simulink model "Diagramas de bloques de un reactor quimico"  (R2018a)
settings: Solver=VariableStepAuto  StartTime=0.0  StopTime=500  RelTol=1e-3
settings Model: Creator=Paulo  LastModifiedBy=Paulo

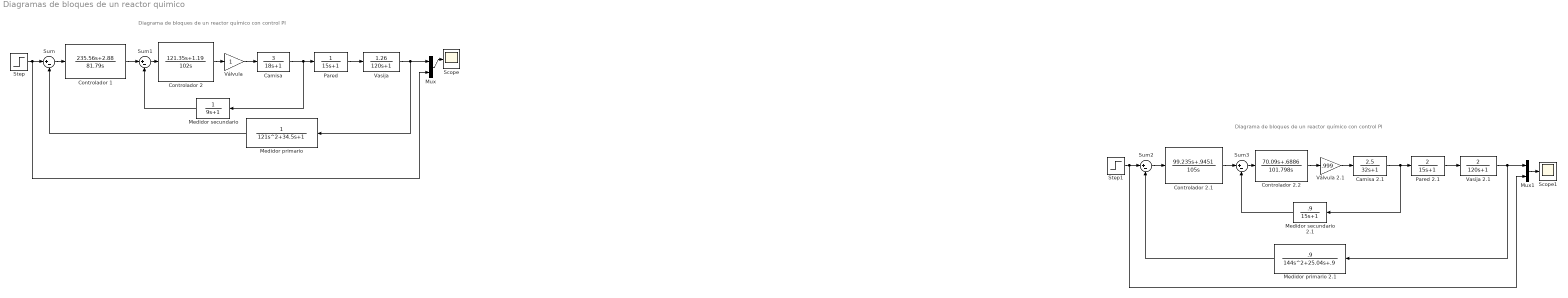
== system Diagramas de bloques de un reactor quimico ==
  note: Diagrama de bloques de un reactor químico con control PI
  note: Diagrama de bloques de un reactor químico con control PI
  Camisa : TransferFcn  Numerator=[3]  Denominator=[18 1]
  Camisa 2.1 : TransferFcn  Numerator=[2.5]  Denominator=[32 1]
  Controlador 1 : TransferFcn  Numerator=[235.56 2.88]  Denominator=[81.79 0]
  Controlador 2 : TransferFcn  Numerator=[121.35 1.19]  Denominator=[102 0]
  "Controlador 2.1 " : TransferFcn  Numerator=[99.235 .9451]  Denominator=[105 0]
  Controlador 2.2 : TransferFcn  Numerator=[70.09 .6886]  Denominator=[101.798 0]
  Medidor primario : TransferFcn  Denominator=[121 34.5 1]
  Medidor primario 2.1 : TransferFcn  Numerator=[.9]  Denominator=[144 25.04 .9]
  Medidor secundario : TransferFcn  Denominator=[9 1]
  Medidor secundario 2.1 : TransferFcn  Numerator=[.9]  Denominator=[15 1]
  Mux : Mux  Inputs=2
  Mux1 : Mux  Inputs=2
  Pared : TransferFcn  Denominator=[15 1]
  Pared 2.1 : TransferFcn  Numerator=[2]  Denominator=[15 1]
  Scope : Scope
  Scope1 : Scope
  Step : Step  Time=0  SampleTime=0
  Step1 : Step  Time=0  SampleTime=0
  Sum{,1..3} (4 alike) : Sum  Inputs=|+-
  Vasija : TransferFcn  Numerator=[1.26]  Denominator=[120 1]
  Vasija 2.1 : TransferFcn  Numerator=[2]  Denominator=[120 1]
  Válvula : Gain
  Válvula 2.1 : Gain  Gain=.999
  wires:
  Step/1 -> Sum/1, Mux/2
  Sum/1 -> Controlador 1/1
  Camisa/1 -> Medidor secundario/1, Pared/1
  Medidor secundario/1 -> Sum1/2
  Válvula/1 -> Camisa/1
  Pared/1 -> Vasija/1
  Vasija/1 -> Mux/1, Medidor primario/1
  Medidor primario/1 -> Sum/2
  Mux/1 -> Scope/1
  Controlador 1/1 -> Sum1/1
  Sum1/1 -> Controlador 2/1
  Controlador 2/1 -> Válvula/1
  Mux1/1 -> Scope1/1
  Camisa 2.1/1 -> Medidor secundario 2.1/1, Pared 2.1/1
  Medidor primario 2.1/1 -> Sum2/2
  Medidor secundario 2.1/1 -> Sum3/2
  Vasija 2.1/1 -> Mux1/1, Medidor primario 2.1/1
  Step1/1 -> Sum2/1, Mux1/2
  Pared 2.1/1 -> Vasija 2.1/1
  Válvula 2.1/1 -> Camisa 2.1/1
  Controlador 2.2/1 -> Válvula 2.1/1
  Sum3/1 -> Controlador 2.2/1
  Sum2/1 -> "Controlador 2.1 "/1
  "Controlador 2.1 "/1 -> Sum3/1
